simulink model "Lab_1_part_1_7"  (R2019b)
settings: Solver=VariableStepAuto  StartTime=0.0  StopTime=10.0  RelTol=1e-3
libraries: commrflib2 x1
settings Model: Creator=mikewang  LastModifiedBy=mikewang

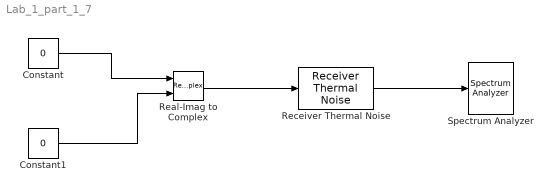
== system Lab_1_part_1_7 ==
  Constant : Constant  Value=0  SampleTime=1e-6
  Constant1 : Constant  Value=0  SampleTime=1e-6
  Real-Imag to Complex : RealImagToComplex
  Receiver Thermal Noise : commrflib2/Receiver Thermal Noise  method=Noise temperature  ntemp=290  nfigure=3.0103  nfactor=2  add290KAntennaNoise=off  seed=randseed
      settings: SourceProductName=Communications Toolbox  SourceProductBaseCode=CM
  Spectrum Analyzer : SpectrumAnalyzer
  wires:
  Constant/1 -> Real-Imag to Complex/1
  Constant1/1 -> Real-Imag to Complex/2
  Real-Imag to Complex/1 -> Receiver Thermal Noise/1
  Receiver Thermal Noise/1 -> Spectrum Analyzer/1
